simulink model "ese1"  (R2021a)
settings: Solver=ode1  StartTime=0.0  StopTime=500  FixedStep=1/1000  RelTol=1e-3
libraries: dspxfrm3 x2, eeGeneralControl x1
settings Model: Creator=giulio  LastModifiedBy=giulio

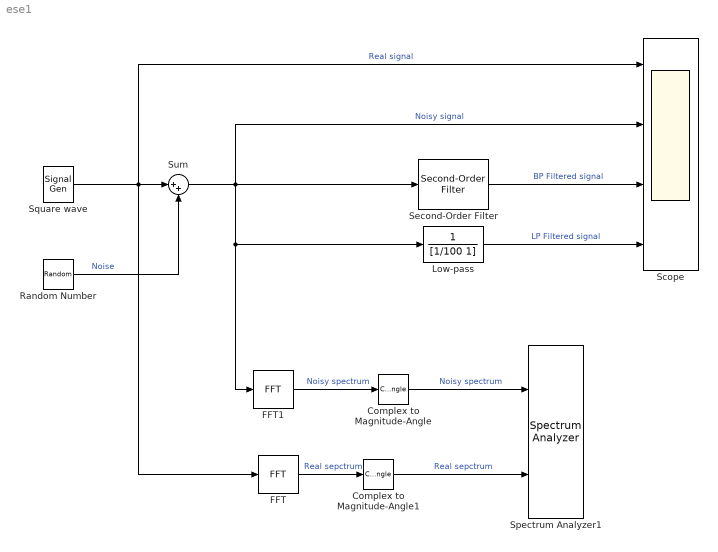
== system ese1 ==
  Complex to Magnitude-Angle : ComplexToMagnitudeAngle  Output=Magnitude
  Complex to Magnitude-Angle1 : ComplexToMagnitudeAngle  Output=Magnitude
  FFT : dspxfrm3/FFT  FFTImplementation=Auto  CompMethod=Table lookup  TableOpt=NEW  TableOptActive=Speed  BitRevOrder=off  Normalize=off  InheritFFTLength=on  FFTLength=64  WrapInput=on  roundingMode=Floor  overflowMode=off  firstCoeffDataTypeStr=Inherit: Same word length as input  firstCoeffLastDataTypeStr=Inherit: Same word length as input  outputMin=[]  outputMax=[]
  FFT1 : dspxfrm3/FFT  FFTImplementation=Auto  CompMethod=Table lookup  TableOpt=NEW  TableOptActive=Speed  BitRevOrder=off  Normalize=off  InheritFFTLength=on  FFTLength=64  WrapInput=on  roundingMode=Floor  overflowMode=off  firstCoeffDataTypeStr=Inherit: Same word length as input  firstCoeffLastDataTypeStr=Inherit: Same word length as input  outputMin=[]  outputMax=[]
  Low-pass : TransferFcn  Denominator=[1/100 1]  ParameterTunability=Optimized
  Random Number : RandomNumber  Variance=0.1  SampleTime=0.001
  Scope : Scope  NumInputPorts=4
  Second-Order Filter : eeGeneralControl/Second-Order Filter  FilterType=Band-pass  fn=10  Zeta=0.5  Ts=-1  A0=0  Ph0=0  f0=0  b0=0
      settings: SourceProductBaseCode=PS
  Spectrum Analyzer1 : SpectrumAnalyzer  NumInputPorts=2
  Square wave : SignalGenerator  WaveForm=square  Frequency=10
  Sum : Sum  Inputs=|++
  wires:
  Square wave/1 -> Scope/1, FFT/1, Sum/1  "Real signal"
  Random Number/1 -> Sum/2  "Noise"
  Sum/1 -> Low-pass/1, FFT1/1, Second-Order Filter/1, Scope/2  "Noisy signal"
  FFT1/1 -> Complex to Magnitude-Angle/1  "Noisy spectrum"
  FFT/1 -> Complex to Magnitude-Angle1/1  "Real sepctrum"
  Second-Order Filter/1 -> Scope/3  "BP Filtered signal"
  Low-pass/1 -> Scope/4  "LP Filtered signal"
  Complex to Magnitude-Angle/1 -> Spectrum Analyzer1/1  "Noisy spectrum"
  Complex to Magnitude-Angle1/1 -> Spectrum Analyzer1/2  "Real sepctrum"
